simulink model "MODEM_ASK"  (R2020a)
settings: Solver=FixedStepDiscrete  StartTime=0.0  StopTime=750  FixedStep=0.001  RelTol=1e-3
libraries: commrandsrc2 x1, simulink x1, dsparch4 x1, dspsrcs4 x1
settings Model: Creator=Administrateur  LastModifiedBy=J-MENTION
settings DataIOCC: LimitDataPoints=on  SaveFormat=Array  SignalLoggingSaveFormat=ModelDataLogs  ReturnWorkspaceOutputs=off
settings OptimizationCC: ExpressionDepthLimit=2147483647  InitFltsAndDblsToZero=on  LifeSpan=inf
settings DebuggingCC: UnderspecifiedInitializationDetection=Classic  MergeDetectMultiDrivingBlocksExec=none  SolverPrmCheckMsg=warning  FcnCallInpInsideContextMsg=warning  StateNameClashWarn=warning  SFUnexpectedBacktrackingDiag=warning  SFNoUnconditionalDefaultTransitionDiag=warning  SFExecutionAtInitializationDiag=none  ArithmeticOperatorsInVariantConditions=warning
settings HardwareCC: ProdBitPerPointer=32  ProdBitPerSizeT=32  ProdBitPerPtrDiffT=32  ProdLargestAtomicFloat=None  ProdIntDivRoundTo=Undefined  ProdEndianess=Unspecified  ProdWordSize=32  ProdHWDeviceType=32-bit Generic
settings ModelReferenceCC: PropagateSignalLabelsOutOfModel=off
settings SFSimCC: SimUseLocalCustomCode=off  CustomCodeUndefinedFunction=UseInterfaceOnly
settings RTWCC: RTWUseLocalCustomCode=off
settings CodeAppCC: StateflowObjectComments=on
settings GRTTargetCC: TargetLangStandard=C89/C90 (ANSI)  CombineOutputUpdateFcns=off  GRTInterface=on
settings ConfigComp: CovMetricSettings=dw  CovHtmlReporting=on  CovSaveCumulativeToWorkspaceVar=on  CovSaveSingleToWorkspaceVar=on  CovExternalEMLEnable=off

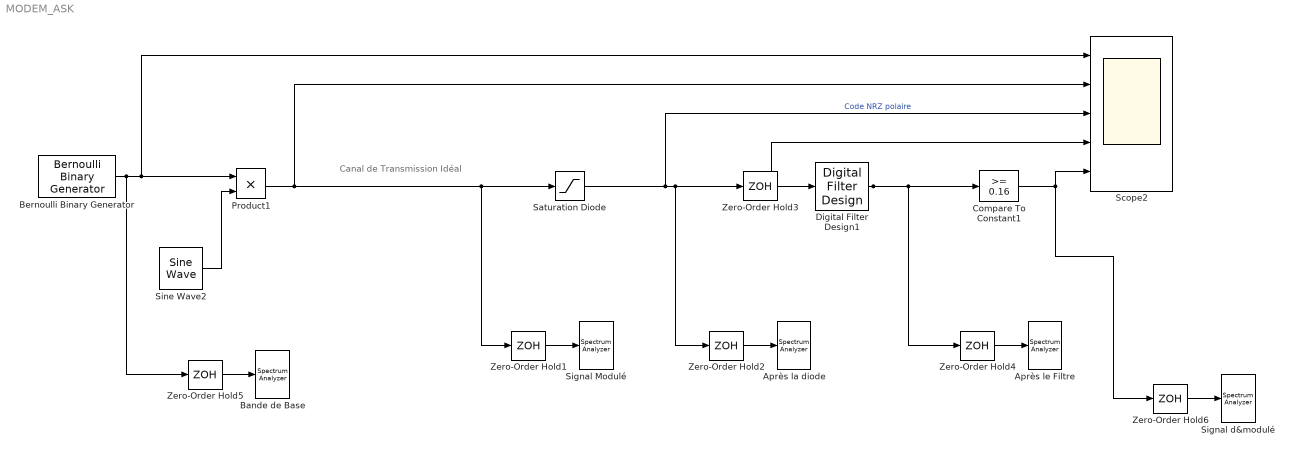
== system MODEM_ASK ==
  note: Canal de Transmission
      | Idéal
  "Après la diode " : SpectrumAnalyzer
  "Après le Filtre " : SpectrumAnalyzer
  "Bande de Base " : SpectrumAnalyzer
  Bernoulli Binary Generator : commrandsrc2/Bernoulli Binary Generator  P=0.5  seed=61  Ts=1  frameBased=off  sampPerFrame=1  orient=off  outDataType=double
      settings: SourceProductBaseCode=CM
  Compare To Constant1 : simulink/Logic and Bit Operations/Compare To Constant  relop=>=  const=0.16  OutDataTypeStr=uint8  ZeroCross=off
  Digital Filter Design1 : dsparch4/Digital Filter Design  mwdsp_browser_bugfix_var=off
  Product1 : Product  RndMeth=Zero
  "Saturation Diode " : Saturate  UpperLimit=2  LowerLimit=0
  Scope2 : Scope  NumInputPorts=5
  "Signal Modulé " : SpectrumAnalyzer
  Signal d&modulé : SpectrumAnalyzer
  Sine Wave2 : dspsrcs4/Sine Wave  Amplitude=1  Frequency=5  Phase=0  SampleMode=Discrete  OutComplex=Real  CompMethod=Trigonometric fcn  TableSize=Speed  SampleTime=1/100  SamplesPerFrame=1  ResetState=Restart at time zero  OutputFrames=on  dataType=double  wordLen=16  udDataType=sfix(16)  fracBitsMode=Best precision  numFracBits=15  OutDataTypeStr=double  LastOutDataTypeStr=double
  Zero-Order Hold{1..2,4,6} (4 alike) : ZeroOrderHold  SampleTime=-1
  Zero-Order Hold3 : ZeroOrderHold  SampleTime=1e-2
  Zero-Order Hold5 : ZeroOrderHold  SampleTime=1/100
  wires:
  Bernoulli Binary Generator/1 -> Zero-Order Hold5/1, Product1/1, Scope2/1
  Sine Wave2/1 -> Product1/2
  Product1/1 -> Zero-Order Hold1/1, "Saturation Diode "/1, Scope2/2
  Digital Filter Design1/1 -> Compare To Constant1/1, Zero-Order Hold4/1, Scope2/4
  Zero-Order Hold3/1 -> Digital Filter Design1/1
  "Saturation Diode "/1 -> Scope2/3, Zero-Order Hold2/1, Zero-Order Hold3/1  "Code NRZ polaire"
  Zero-Order Hold1/1 -> "Signal Modulé "/1
  Zero-Order Hold2/1 -> "Après la diode "/1
  Zero-Order Hold4/1 -> "Après le Filtre "/1
  Zero-Order Hold5/1 -> "Bande de Base "/1
  Zero-Order Hold6/1 -> Signal d&modulé/1
  Compare To Constant1/1 -> Zero-Order Hold6/1, Scope2/5
